simulink model "untitled"  (R2020a)
settings: Solver=VariableStepAuto  StartTime=0.0  StopTime=10  RelTol=1e-3
settings Model: Creator=g-oft  LastModifiedBy=g-oft

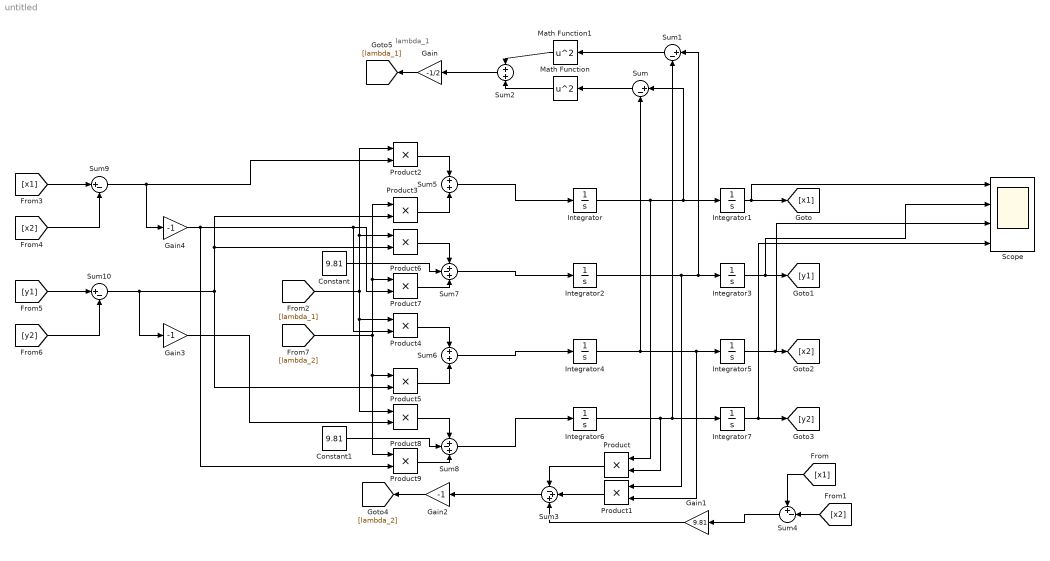
== system untitled ==
  note: lambda_1
  Constant : Constant  Value=9.81
  Constant1 : Constant  Value=9.81
  Gain : Gain  Gain=-1/2
  Gain1 : Gain  Gain=9.81
  Gain2 : Gain  Gain=-1
  Gain3 : Gain  Gain=-1
  Gain4 : Gain  Gain=-1
  Integrator : Integrator  InitialCondition=1
  Integrator1 : Integrator  InitialCondition=5
  Integrator2 : Integrator
  Integrator3 : Integrator  InitialCondition=4
  Integrator4 : Integrator  InitialCondition=1
  Integrator5 : Integrator  InitialCondition=6
  Integrator6 : Integrator
  Integrator7 : Integrator  InitialCondition=4
  Math Function : Math  Operator=square  SaturateOnIntegerOverflow=on
  Math Function1 : Math  Operator=square  SaturateOnIntegerOverflow=on
  Product{,1..9} (10 alike) : Product
  Scope : Scope  NumInputPorts=4
  Sum{,1,9..10} (4 alike) : Sum  Inputs=|+-
  Sum2 : Sum
  Sum3 : Sum  Inputs=-++
  Sum4 : Sum  Inputs=+-|
  Sum5 : Sum
  Sum6 : Sum
  Sum7 : Sum  Inputs=+-+
  Sum8 : Sum  Inputs=+-+
  wires:
  Integrator/1 -> Product/1, Sum/1, Integrator1/1
  Integrator4/1 -> Sum/2, Product1/2, Integrator5/1
  Integrator6/1 -> Product/2, Sum1/2, Integrator7/1
  Integrator2/1 -> Product1/1, Sum1/1, Integrator3/1
  Sum/1 -> Math Function/1
  Sum1/1 -> Math Function1/1
  Math Function1/1 -> Sum2/1
  Math Function/1 -> Sum2/2
  Sum2/1 -> Gain/1
  Product1/1 -> Sum3/2
  Product/1 -> Sum3/1
  Sum4/1 -> Gain1/1
  Gain1/1 -> Sum3/3
  Sum3/1 -> Gain2/1
  Product2/1 -> Sum5/1
  Product3/1 -> Sum5/2
  Product4/1 -> Sum6/1
  Product5/1 -> Sum6/2
  Product6/1 -> Sum7/1
  Constant/1 -> Sum7/2
  Product7/1 -> Sum7/3
  Product9/1 -> Sum8/3
  Product8/1 -> Sum8/1
  Constant1/1 -> Sum8/2
  Sum8/1 -> Integrator6/1
  Sum6/1 -> Integrator4/1
  Sum7/1 -> Integrator2/1
  Sum5/1 -> Integrator/1
  Integrator1/1 -> Scope/1, [x1]
  Integrator3/1 -> Scope/2, [y1]
  Integrator5/1 -> Scope/3, [x2]
  Integrator7/1 -> Scope/4, [y2]
  Gain2/1 -> [lambda_2]
  Gain/1 -> [lambda_1]
  [x1] -> Sum4/1
  [x2] -> Sum4/2
  [lambda_1] -> Product2/1, Product6/1, Product8/1, Product4/1
  [x2] -> Sum9/2
  [x1] -> Sum9/1
  [y1] -> Sum10/1
  [y2] -> Sum10/2
  Sum9/1 -> Gain4/1, Product2/2
  [lambda_2] -> Product3/1, Product7/1, Product9/1, Product5/1
  Sum10/1 -> Gain3/1, Product5/2, Product6/2, Product3/2
  Gain4/1 -> Product9/2, Product7/2, Product4/2
  Gain3/1 -> Product8/2
